simulink model "GlazedSolarCollector_2node"  (R2018b)
settings: Solver=ode45  StartTime=0  StopTime=96*3600  MaxStep=600  RelTol=1e-3  EnableMultiTasking=on
InitFcn:
  | load('DE_TRY2010_13_averageYear')
undefined symbols (not defined in the file): path_carnot
libraries: carnot x11, simulink x2
settings Model: Creator=drhf  LastModifiedBy=drhf
settings DataIOCC: SaveFormat=Array  SignalLoggingSaveFormat=ModelDataLogs
settings OptimizationCC: ExpressionDepthLimit=2147483647  LifeSpan=inf
settings DebuggingCC: UnderspecifiedInitializationDetection=Classic  MergeDetectMultiDrivingBlocksExec=none  SolverPrmCheckMsg=warning  FcnCallInpInsideContextMsg=warning  StateNameClashWarn=warning  SFUnexpectedBacktrackingDiag=warning  SFNoUnconditionalDefaultTransitionDiag=warning  SFExecutionAtInitializationDiag=none
settings HardwareCC: ProdBitPerPointer=32  ProdBitPerSizeT=32  ProdBitPerPtrDiffT=32  ProdLargestAtomicFloat=None  ProdIntDivRoundTo=Undefined  ProdEndianess=Unspecified  ProdWordSize=32  ProdHWDeviceType=32-bit Generic
settings ModelReferenceCC: PropagateSignalLabelsOutOfModel=off
settings SFSimCC: SimUseLocalCustomCode=off
settings RTWCC: RTWUseLocalCustomCode=off
settings CodeAppCC: StateflowObjectComments=on
settings GRTTargetCC: TargetLangStandard=C89/C90 (ANSI)  CombineOutputUpdateFcns=off  GRTInterface=on
settings ConfigComp: CovMetricSettings=dw  CovSaveCumulativeToWorkspaceVar=on  CovSaveSingleToWorkspaceVar=on  CovExternalEMLEnable=off

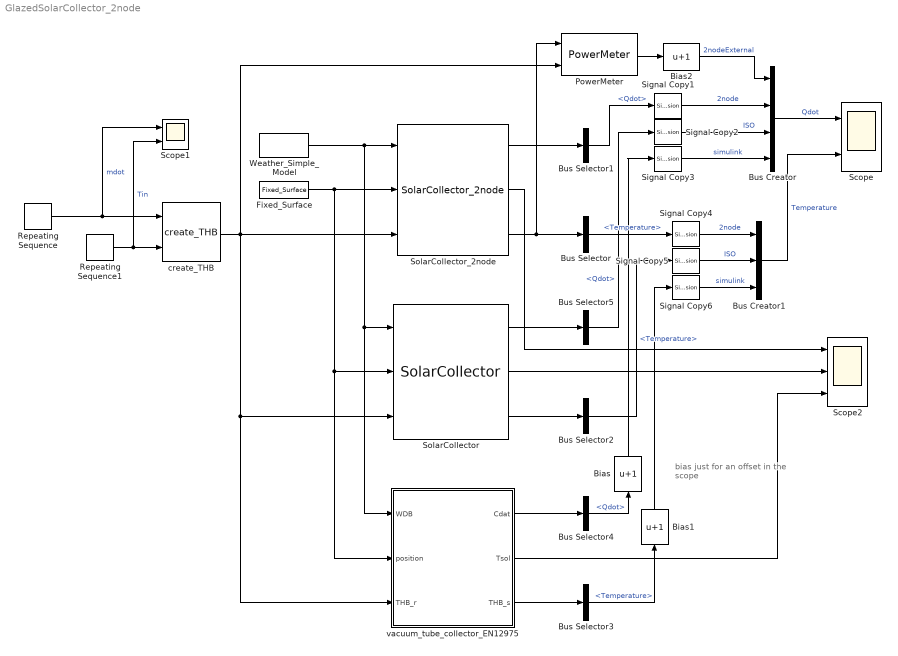
== system GlazedSolarCollector_2node ==
  note: bias just for an
      | offset in the scope
  Bias : Bias  Bias=1
  Bias1 : Bias  Bias=1
  Bias2 : Bias  Bias=1
  Bus Creator : BusCreator  Inputs=4
  Bus Creator1 : BusCreator  Inputs=3
  Bus Selector : BusSelector  OutputSignals=Temperature
  Bus Selector1 : BusSelector  OutputSignals=Qdot
  Bus Selector2 : BusSelector  OutputSignals=Temperature
  Bus Selector3 : BusSelector  OutputSignals=Temperature
  Bus Selector4 : BusSelector  OutputSignals=Qdot
  Bus Selector5 : BusSelector  OutputSignals=Qdot
  Fixed_Surface : carnot/Weather/Fixed_Surface  colangle=30  colazi=0  colrot=0
      settings: SourceProductName=Carnot
  PowerMeter : carnot/Control/PowerMeter
      settings: SourceProductName=Carnot
  Repeating Sequence : simulink/Sources/Repeating Sequence  rep_seq_t=[0 24 36 48 60 100]*3600  rep_seq_y=[126 126 10 126 126 126]/3600
  Repeating Sequence1 : simulink/Sources/Repeating Sequence  rep_seq_t=[0 24 36 48 60 100]*3600  rep_seq_y=[20 20 20 20 5 5]
  Scope : Scope  NumInputPorts=2
  Scope1 : Scope  NumInputPorts=2
  Scope2 : Scope  NumInputPorts=3
  Signal Copy{1..6} (6 alike) : SignalConversion  OverrideOpt=off
  SolarCollector : carnot/Source/Solar_Thermal/SolarCollector  t0=20  Ncollector=2  PathName=fullfile(path_carnot('libsl'), 'Source', 'Solar_Thermal', 'SolarCollector', 'parameter_set')  FileName='DefaultCollector.mat'  userPath=off  userParam=off  acol=3.5  len=0.1  fta=0.7  c1=1.1  c2=0.001  c3=0  c4=0  c5=5000  c6=0  KbAngles=[0 5 10 15 20 25 30 35 40 45 50 55 60 65 70 75 80 85 90]  KbL=[1 1 0.9999 0.9996 0.9991 0.9982 0.9965 0.9935 0.9886 0.9807 0.9678 0.9473 0.9148 0.8638 0.7846 0.6644 0.4907 0.2599 0]  KbT=[1 1 1 1 1 1 1 1 1 1 1 0.875 0.75 0.625 0.5 0.375 0.25 0.125 0]  Kd=0.92  dplin=10  dpqua=10  SensorTimeConstant=10
      settings: SourceProductName=Carnot
  SolarCollector_2node : carnot/Source/Solar_Thermal/SolarCollector_2node  t0=20  Ncollector=2  PathName=fullfile(path_carnot('libsl'), 'Source', 'Solar_Thermal', 'SolarCollector_2node', 'parameter_set')  FileName='DefaultCollector.mat'  userPath=off  userParam=off  acol=3.5  len=0.1  fta=0.7  c1=1.1  c2=0.001  c3=0  c4=0  c5=5000  c6=0  KbAngles=[0 5 10 15 20 25 30 35 40 45 50 55 60 65 70 75 80 85 90]  KbL=[1 1 0.9999 0.9996 0.9991 0.9982 0.9965 0.9935 0.9886 0.9807 0.9678 0.9473 0.9148 0.8638 0.7846 0.6644 0.4907 0.2599 0]  KbT=[1 1 1 1 1 1 1 1 1 1 1 0.875 0.75 0.625 0.5 0.375 0.25 0.125 0]  Kd=0.92  dplin=10  dpqua=10  SensorTimeConstant=10
      settings: SourceProductName=Carnot
  Weather_Simple_Model : carnot/Weather/Weather_Simple_Model  Ibn=900  Idg=100  tamb=5  deltaTsky=-6  rh=50  precip="10e-3/24/3600           % 10 mm in 24 h"  cloud=0.125  p=1013e2  vw=1  wdir=270  lat=60  colangle=0  colazi=0  colrot=0
      settings: SourceProductName=Carnot
  create_THB : carnot/Source/Simple/create_THB  p=1e5  fluid=Water  mix=0  mix2=0  mix3=0  dia=0  hgt=0  mID=No Pressure Drop
      settings: SourceProductName=Carnot
  vacuum_tube_collector_EN12975 : Subsystem  mask(Solar Thermal Collector){t0=20, Ncollector=2, PathName=fullfile(path_carnot('libsl'), 'Source', 'Solar_Thermal', 'SolarCollector', 'parameter_set'), FileName='DefaultCollector.mat', userPath=off, userParam=off, acol=3.5, len=0.1, fta=0.7, c1=1.1, c2=0.001, c3=0, c4=0, c5=5000, c6=0, KbAngles=[0 5 10 15 20 25 30 35 40 45 50 55 60 65 70 75 80 85 90], KbL=[1 1 0.9999 0.9996 0.9991 0.9982 0.9965 0.9935 0.9886 0.9807 0.9678 0.9473 0.9148 0.8638 0.7846 0.6644 0.4907 0.2599 0], KbT=[1 1 1 1 1 1 1 1 1 1 1 0.875 0.75 0.625 0.5 0.375 0.25 0.125 0], Kd=0.92, dplin=10, dpqua=10, SensorTimeConstant=10}
      mask prompts: t0 "Initial temperature [°C]"; Ncollector "Number of collectors in parallel"; PathName "Path"; FileName "Parameter set"; userPath "Edit path and name of parameter set"; userParam "User defined parameters"; acol "A: surface  of one collector module in m²"; len "Length between collector inlet and outlet in m"; fta "Fin Efficiency * Transmission * Absorption (F'(tau alfa))"; c1 "c1 : heat loss coefficient at (Tm-Ta)=0  [W/(m²*K)]"; c2 "c2: temperature dependence of the heat loss coefficient [W/(m*K)²]"; c3 "c3 : wind speed dependence of the heat loss coefficient [J/(m³K)]"; c4 "c4 : sky temperature dependence of the heat loss coefficient [W/(m²K)]"; c5 "c5 : effective thermal capacity [J/(m²K)]"; c6 "c6 : wind dependence in the zero loss efficiency [s/m]"; KbAngles "Kb: angles for longitudinal and transversal IAM [degree]"; KbL "KbL: values for longitudinal incidence angle modifier (0..1)"; KbT "KbT: values for transversal incidence angle modifier (0..1)"; Kd "Kd : Incidence angle modifier diffuse radiation"; dplin "lin: linear pressure drop in Pa/(kg/s)"; dpqua "qua: quadratic pressure drop in Pa/(kg/s)²"; SensorTimeConstant "time constant of sensor [s]"
      mask help: Dynamic 1-node solar thermal collector model according to ISO 9806 standard. Collector optics use a lookup table for the incidence angle modifier. Especially tube collectors have asymmetric IAM and require a geometry dependancy.
      mask init:
      | % callback to set parameters of model
      | [ok, param] = CarnotCallbacks_CollectorEN12975Conf('SetParameters',gcbh,PathName,FileName);
      mask Help: web(fullfile(path_carnot('help'),'collector_en12975.html'),'-helpbrowser')
      mask TypeOptions t0: T_Sensor/t0 | solar_collector_basic/tini
      mask TypeOptions Ncollector: Ncollector/Value | Gain1/Gain | Gain2/Gain
      mask Callback userPath: [ok, param] = CarnotCallbacks_CollectorEN12975Conf('UserEdit',gcbh);
      mask Callback userParam: [ok, param] = CarnotCallbacks_CollectorEN12975Conf('UserEdit',gcbh);
      mask TypeOptions acol: solar_collector_basic/acol | Acol/Value
      mask TypeOptions len: Pressure_Drop_Collector/len
      mask TypeOptions fta: IAM_Table_KbL_KbT/fta
      mask TypeOptions c1: solar_collector_basic/c1
      mask TypeOptions c2: solar_collector_basic/c2
      mask TypeOptions c3: solar_collector_basic/c3
      mask TypeOptions c4: solar_collector_basic/c4
      mask TypeOptions c5: solar_collector_basic/c5
      mask TypeOptions c6: solar_collector_basic/c6
      mask TypeOptions KbAngles: IAM_Table_KbL_KbT/kblangle | IAM_Table_KbL_KbT/kbtangle
      mask TypeOptions KbL: IAM_Table_KbL_KbT/KbL
      mask TypeOptions KbT: IAM_Table_KbL_KbT/KbT
      mask TypeOptions Kd: IAM_Table_KbL_KbT/Kd
      mask TypeOptions dplin: Pressure_Drop_Collector/lin
      mask TypeOptions dpqua: Pressure_Drop_Collector/qua
      mask TypeOptions SensorTimeConstant: T_Sensor/tc
      mask DialogControl ParameterGroupVar Prompt: Picking a parameter set
      mask DialogControl Control2 Prompt: Carnot public data
      mask DialogControl Control2 Callback: [ok, file] = CarnotCallbacks_CollectorEN12975Conf('GetFilename',gcbh,'public');
      mask DialogControl Control3 Prompt: Carnot internal data
      mask DialogControl Control3 Callback: [ok, file] = CarnotCallbacks_CollectorEN12975Conf('GetFilename',gcbh,'internal');
      mask DialogControl Control4 Prompt: Selected path
      mask DialogControl Control4 Callback: [ok, file] = CarnotCallbacks_CollectorEN12975Conf('GetFilename',gcbh,'selected');
      mask DialogControl Container7 Prompt: Geometry
      mask DialogControl Container8 Prompt: Coll.Params
      mask DialogControl Container9 Prompt: Optics
      mask DialogControl Container10 Prompt: Hydraulic
      mask DialogControl Container11 Prompt: Sensors
      mask DialogControl Control5 Prompt: Save in Carnot interal data
      mask DialogControl Control5 Callback: [ok, param] = CarnotCallbacks_CollectorEN12975Conf('SaveFilename',gcbh,'internal','COL');
      mask DialogControl Control6 Prompt: Save in seleced path
      mask DialogControl Control6 Callback: [ok, param] = CarnotCallbacks_CollectorEN12975Conf('SaveFilename',gcbh,'selected','COL');
      mask Display:
      | % user defined picture file
      | picfile = fullfile(path_carnot('intlibsl'), ...
      |     'Source','Solar_Thermal','SolarCollector','parameter_set', ...
      |      'Collector_CONF.jpg');
      | 
      | pic = false;
      | 
      | % show internal picture if defined
      | if ~BlockIsInCarnotLibrary    % if not located in library any more
      |     if exist(picfile)
      |         image(imread(picfile), [0.2, 0, 0.6, 1])
      |         set_param(gcb, 'BackgroundColor', 'White')
      |         pic = true;
      |     end
      | end
      | 
      | if ~pic    % show public picture
      |     disp('Solar Thermal\nCollector\n\nISO 9806')
      |     set_param(gcb, 'BackgroundColor', 'Yellow')
      | end
  wires:
  Weather_Simple_Model/1 -> vacuum_tube_collector_EN12975/1(WDB), SolarCollector/1, SolarCollector_2node/1
  create_THB/1 -> SolarCollector_2node/3, SolarCollector/3, vacuum_tube_collector_EN12975/3(THB_r), PowerMeter/2
  Fixed_Surface/1 -> SolarCollector_2node/2, SolarCollector/2, vacuum_tube_collector_EN12975/2(position)
  SolarCollector_2node/1 -> Bus Selector1/1
  Bus Selector1/1 -> Signal Copy1/1  "<Qdot>"
  SolarCollector_2node/3 -> PowerMeter/1, Bus Selector/1
  SolarCollector_2node/2 -> Scope2/1
  Bus Creator1/1 -> Scope/2  "Temperature"
  vacuum_tube_collector_EN12975/3(THB_s) -> Bus Selector3/1
  vacuum_tube_collector_EN12975/1(Cdat) -> Bus Selector4/1
  vacuum_tube_collector_EN12975/2(Tsol) -> Scope2/3
  Bus Selector4/1 -> Bias/1  "<Qdot>"
  Bus Creator/1 -> Scope/1  "Qdot"
  SolarCollector/1 -> Bus Selector5/1
  Bus Selector5/1 -> Signal Copy2/1  "<Qdot>"
  SolarCollector/3 -> Bus Selector2/1
  SolarCollector/2 -> Scope2/2
  Signal Copy1/1 -> Bus Creator/2  "2node"
  Signal Copy2/1 -> Bus Creator/3  "ISO"
  Signal Copy3/1 -> Bus Creator/4  "simulink"
  Signal Copy6/1 -> Bus Creator1/3  "simulink"
  Signal Copy5/1 -> Bus Creator1/2  "ISO"
  Signal Copy4/1 -> Bus Creator1/1  "2node"
  Bus Selector/1 -> Signal Copy4/1  "<Temperature>"
  Bus Selector2/1 -> Signal Copy5/1  "<Temperature>"
  Bus Selector3/1 -> Bias1/1  "<Temperature>"
  Bias/1 -> Signal Copy3/1
  Repeating Sequence1/1 -> Scope1/2, create_THB/2  "Tin"
  Repeating Sequence/1 -> Scope1/1, create_THB/1  "mdot"
  PowerMeter/1 -> Bias2/1
  Bias1/1 -> Signal Copy6/1
  Bias2/1 -> Bus Creator/1  "2nodeExternal"

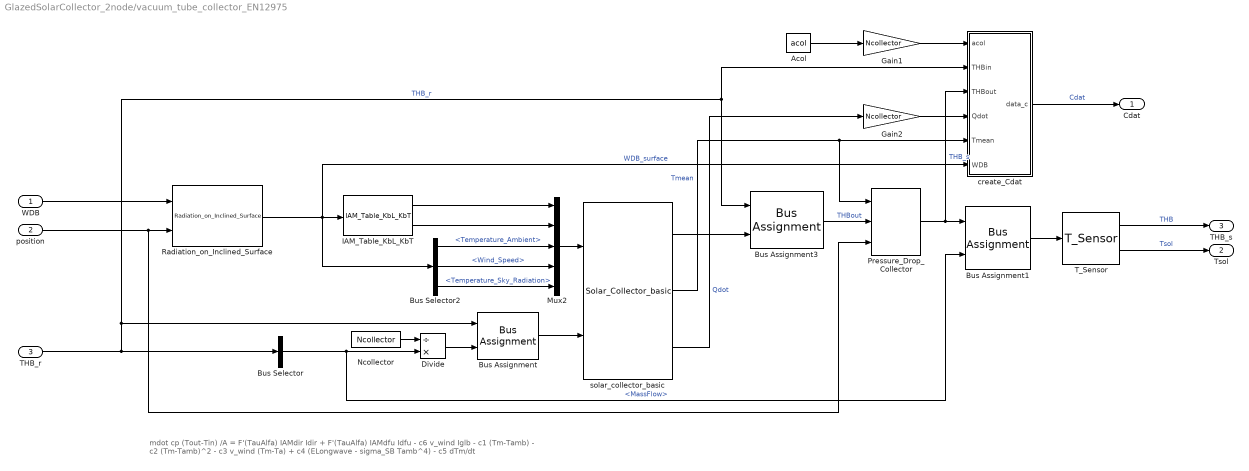
== system GlazedSolarCollector_2node/vacuum_tube_collector_EN12975 ==
  note: mdot cp (Tout-Tin) /A = F'(TauAlfa) IAMdir Idir + F'(TauAlfa) IAMdfu Idfu - c6 v_wind Iglb - c1 (Tm-Tamb) - c2 (Tm-Tamb)^2 - c3 v_wind (Tm-Ta) + c4 (ELongwave - sigma_SB Tamb^4) - c5 dTm/dt
  WDB : Inport
  position : Inport  Port=2
  THB_r : Inport  Port=3
  Acol : Constant  Value=acol
  Bus Assignment : BusAssignment  AssignedSignals=MassFlow
  Bus Assignment1 : BusAssignment  AssignedSignals=MassFlow
  Bus Assignment3 : BusAssignment  AssignedSignals=Temperature
  Bus Selector : BusSelector  OutputSignals=MassFlow
  Bus Selector2 : BusSelector  OutputSignals=Temperature_Ambient,Wind_Speed,Temperature_Sky_Radiation
  Divide : Product  Inputs=/*
  Gain1 : Gain  Gain=Ncollector
  Gain2 : Gain  Gain=Ncollector
  IAM_Table_KbL_KbT : carnot/Source/Solar_Thermal/IncidenceAngleModifier/IAM_Table_KbL_KbT  fta=fta  kblangle=KbAngles  KbL=KbL  kbtangle=KbAngles  KbT=KbT  Kd=Kd
      settings: SourceProductName=Carnot
  Mux2 : Mux  Inputs=5
  Ncollector : Constant  Value=Ncollector
  Pressure_Drop_Collector : carnot/Basic/Pressure_Drop/Pressure_Drop_Collector  len=len  lin=dplin  qua=dpqua
      settings: SourceProductName=Carnot
  Radiation_on_Inclined_Surface : carnot/Weather/Radiation_on_Inclined_Surface  sky=Perez 1990  reflect=0.2
      settings: SourceProductName=Carnot
  T_Sensor : carnot/Control/T_Sensor  tc=SensorTimeConstant  t0=t0
      settings: SourceProductName=Carnot
  create_Cdat : Subsystem
  solar_collector_basic : carnot/Basic/Thermal_Models/Solar_Collector_basic  acol=acol  c1=c1  c2=c2  c3=c3  c4=c4  c5=c5  c6=c6  tini=t0
      settings: SourceProductName=Carnot
  Cdat : Outport  VectorParamsAs1DForOutWhenUnconnected=off
  Tsol : Outport  Port=2  VectorParamsAs1DForOutWhenUnconnected=off
  THB_s : Outport  Port=3  VectorParamsAs1DForOutWhenUnconnected=off
  wires:
  T_Sensor/1 -> THB_s/1  "THB"
  T_Sensor/2 -> Tsol/1  "Tsol"
  Divide/1 -> Bus Assignment/2
  Ncollector/1 -> Divide/1
  Bus Assignment/1 -> solar_collector_basic/2
  WDB/1 -> Radiation_on_Inclined_Surface/1
  solar_collector_basic/3 -> Gain2/1  "Qdot"
  Bus Assignment3/1 -> Pressure_Drop_Collector/2  "THBout"
  THB_r/1 -> Bus Selector/1, create_Cdat/2(THBin), Bus Assignment3/1, Bus Assignment/1  "THB_r"
  solar_collector_basic/1 -> Bus Assignment3/2
  solar_collector_basic/2 -> create_Cdat/5(Tmean), Pressure_Drop_Collector/1  "Tmean"
  IAM_Table_KbL_KbT/2 -> Mux2/2
  Bus Selector2/3 -> Mux2/5  "<Temperature_Sky_Radiation>"
  create_Cdat/1(data_c) -> Cdat/1  "Cdat"
  Radiation_on_Inclined_Surface/1 -> create_Cdat/6(WDB), Bus Selector2/1, IAM_Table_KbL_KbT/1  "WDB_surface"
  Mux2/1 -> solar_collector_basic/1
  Bus Selector2/1 -> Mux2/3  "<Temperature_Ambient>"
  Pressure_Drop_Collector/1 -> Bus Assignment1/1, create_Cdat/3(THBout)  "THB_s"
  IAM_Table_KbL_KbT/1 -> Mux2/1
  Bus Selector2/2 -> Mux2/4  "<Wind_Speed>"
  position/1 -> Pressure_Drop_Collector/3, Radiation_on_Inclined_Surface/2
  Acol/1 -> Gain1/1
  Bus Selector/1 -> Bus Assignment1/2, Divide/2  "<MassFlow>"
  Gain1/1 -> create_Cdat/1(acol)
  Gain2/1 -> create_Cdat/4(Qdot)
  Bus Assignment1/1 -> T_Sensor/1

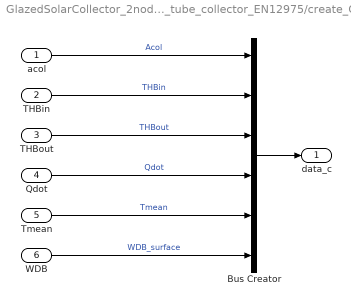
== system GlazedSolarCollector_2node/vacuum_tube_collector_EN12975/create_Cdat ==
  acol : Inport
  THBin : Inport  Port=2
  THBout : Inport  Port=3
  Qdot : Inport  Port=4
  Tmean : Inport  Port=5
  WDB : Inport  Port=6
  Bus Creator : BusCreator  Inputs=6
  data_c : Outport  VectorParamsAs1DForOutWhenUnconnected=off
  wires:
  Tmean/1 -> Bus Creator/5  "Tmean"
  Qdot/1 -> Bus Creator/4  "Qdot"
  Bus Creator/1 -> data_c/1
  WDB/1 -> Bus Creator/6  "WDB_surface"
  THBout/1 -> Bus Creator/3  "THBout"
  THBin/1 -> Bus Creator/2  "THBin"
  acol/1 -> Bus Creator/1  "Acol"
